simulink model "sf_ladder_logic_scheduler"  (R2017b)
settings: Solver=FixedStepDiscrete  StartTime=0.0  StopTime=10  RelTol=1e-3  EnableMultiTasking=on
model workspace (MAT data in the model file):
  deltat = 0.001
settings Model: Creator=The MathWorks, Inc.  LastModifiedBy=The MathWorks, Inc.
settings SolverCC: InsertRTBMode=Auto
settings DataIOCC: LimitDataPoints=on  SaveFormat=Array
settings OptimizationCC: ExpressionDepthLimit=2147483647  InitFltsAndDblsToZero=on  LifeSpan=inf
settings DebuggingCC: SaveWithParameterizedLinksMsg=none  UnderspecifiedInitializationDetection=Classic  MergeDetectMultiDrivingBlocksExec=none  SignalResolutionControl=TryResolveAllWithWarning  SolverPrmCheckMsg=warning  InheritedTsInSrcMsg=none  MultiTaskDSMMsg=warning  MultiTaskCondExecSysMsg=none  FcnCallInpInsideContextMsg=warning  StateNameClashWarn=warning  StrictBusMsg=None  SFUnexpectedBacktrackingDiag=warning  SFNoUnconditionalDefaultTransitionDiag=warning  SFExecutionAtInitializationDiag=none
settings HardwareCC: ProdBitPerPointer=32  ProdBitPerSizeT=32  ProdBitPerPtrDiffT=32  ProdLargestAtomicFloat=None  ProdIntDivRoundTo=Undefined  ProdEndianess=Unspecified  ProdWordSize=32  ProdHWDeviceType=32-bit Generic
settings ModelReferenceCC: PropagateSignalLabelsOutOfModel=off
settings SFSimCC: SFSimEcho=off  SimParseCustomCode=off
settings CodeAppCC: StateflowObjectComments=on
settings GRTTargetCC: TargetFcnLib=ansi_tfl_tmw.mat  TargetLangStandard=C89/C90 (ANSI)  GeneratePreprocessorConditionals=Disable all  CombineOutputUpdateFcns=off  GRTInterface=on
settings ConfigComp: CovMetricSettings=dw  CovHtmlReporting=on  CovSaveCumulativeToWorkspaceVar=on  CovSaveSingleToWorkspaceVar=on  CovExternalEMLEnable=off  CovSFcnEnable=off

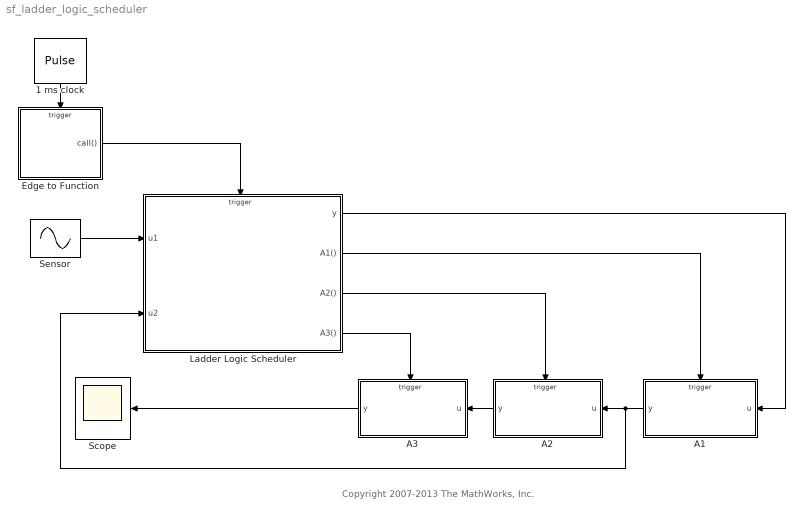
== system sf_ladder_logic_scheduler ==
  note: Copyright 2007-2013 The MathWorks, Inc.
  1 ms clock : DiscretePulseGenerator  PulseType=Time based  Period=0.001  PulseWidth=10
  A1 : Subsystem  TreatAsAtomicUnit=on
  A2 : Subsystem  TreatAsAtomicUnit=on
  A3 : Subsystem  TreatAsAtomicUnit=on
  "Edge to Function " : Stateflow chart  TreatAsAtomicUnit=on
  Ladder Logic Scheduler : Stateflow chart  TreatAsAtomicUnit=on
  Scope : Scope
  Sensor : Sin  Frequency=40  Phase=-pi/8
  wires:
  Ladder Logic Scheduler/1(y) -> A1/1(u)
  Ladder Logic Scheduler/2(A1()) -> A1/Trigger
  Ladder Logic Scheduler/3(A2()) -> A2/Trigger
  Ladder Logic Scheduler/4(A3()) -> A3/Trigger
  A1/1(y) -> Ladder Logic Scheduler/2(u2), A2/1(u)
  A2/1(y) -> A3/1(u)
  Sensor/1 -> Ladder Logic Scheduler/1(u1)
  1 ms clock/1 -> "Edge to Function "/Trigger
  "Edge to Function "/1(call()) -> Ladder Logic Scheduler/Trigger
  A3/1(y) -> Scope/1

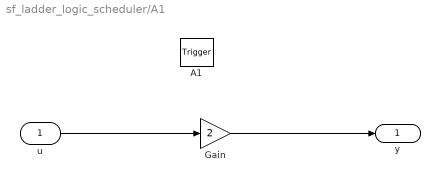
== system sf_ladder_logic_scheduler/A1 ==
  u : Inport
  A1 : TriggerPort  TriggerType=function-call  VariantControl=(inherit)
  Gain : Gain  Gain=2
  y : Outport
  wires:
  u/1 -> Gain/1
  Gain/1 -> y/1

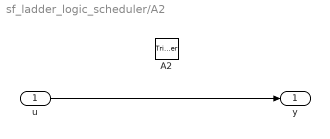
== system sf_ladder_logic_scheduler/A2 ==
  u : Inport
  A2 : TriggerPort  TriggerType=function-call  VariantControl=(inherit)
  y : Outport  InitialOutput=0
  wires:
  u/1 -> y/1

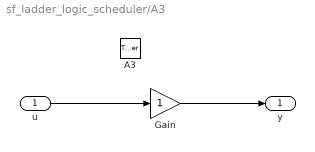
== system sf_ladder_logic_scheduler/A3 ==
  u : Inport
  A3 : TriggerPort  TriggerType=function-call  VariantControl=(inherit)
  Gain : Gain
  y : Outport
  wires:
  u/1 -> Gain/1
  Gain/1 -> y/1

== stateflow chart sf_ladder_logic_scheduler/Ladder Logic Scheduler ==
  note: Sequencing
      | Ladder Logic
  (default) -> (junction 12) : {y=u1}
  (junction 12) -> (junction 13) [order 1] : [u1>0]
  (junction 12) -> (junction 14) [order 2]
  (junction 13) -> (junction 14) : {send(A1)}
  (junction 14) -> (junction 15) [order 1] : [u2 >= 0]
  (junction 14) -> (junction 16) [order 2]
  (junction 15) -> (junction 16) : {send(A2)}
  (junction 16) -> (junction 17) [order 1] : [(u1>0) && (u2>0)]
  (junction 16) -> (junction 18) [order 2]
  (junction 17) -> (junction 18) : {send(A3)}
  data: y output double; u1 input; u2 input
  events: A1 output FUNCTION_CALL_EVENT; A2 output FUNCTION_CALL_EVENT; A3 output FUNCTION_CALL_EVENT; call input FUNCTION_CALL_EVENT

== stateflow chart sf_ladder_logic_scheduler/Edge to Function  ==
  (default) -> (junction 2) : {call;}
  events: edge input RISING_EDGE_EVENT; call output FUNCTION_CALL_EVENT
